simulink model "Sim2"  (R2014a)
settings: Solver=ode45  StartTime=0.0  StopTime=10.0  RelTol=1e-3
settings Model: Creator=OCAC  LastModifiedBy=OCAC

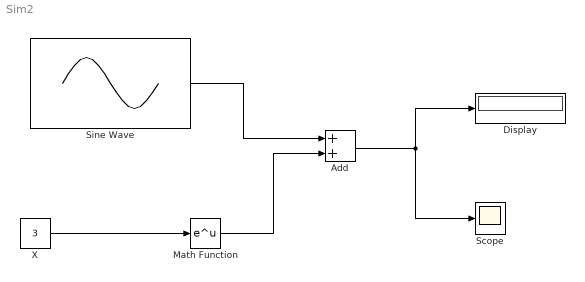
== system Sim2 ==
  Add : Sum
  Display : Display
  Math Function : Math  SaturateOnIntegerOverflow=on
  Scope : Scope
  Sine Wave : Sin  SampleTime=0
  "X " : Constant  Value=3
  wires:
  "X "/1 -> Math Function/1
  Math Function/1 -> Add/2
  Sine Wave/1 -> Add/1
  Add/1 -> Scope/1, Display/1
